simulink model "Ser_RLC_Sys"  (R2015a)
settings: Solver=ode23  StartTime=0.0  StopTime=0.01  RelTol=1e-3
settings Model: Creator=Kunal  LastModifiedBy=Kunal
settings SolverCC: AutoInsertRateTranBlk=on

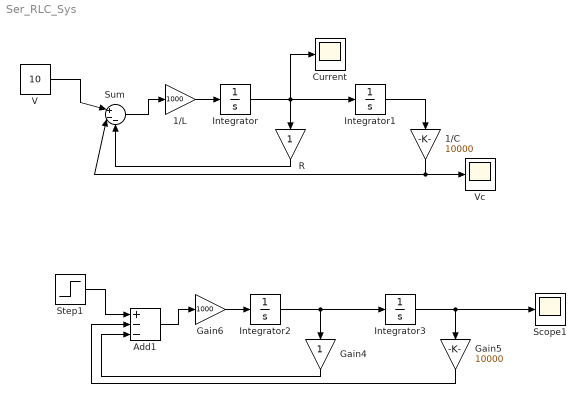
== system Ser_RLC_Sys ==
  1/C : Gain  Gain=10000
  1/L : Gain  Gain=1000
  Add1 : Sum  Inputs=+--
  Current : Scope
      settings: SaveName=ScopeData2  MaxDataPoints=5000000
  Gain4 : Gain
  Gain5 : Gain  Gain=10000
  Gain6 : Gain  Gain=1000
  Integrator{,1..3} (4 alike) : Integrator
  R : Gain
  Scope1 : Scope
  Step1 : Step  Time=0  After=10  SampleTime=0
  Sum : Sum  Inputs=|+--
  V : Constant  Value=10
  Vc : Scope
      settings: MaxDataPoints=5000000
  wires:
  Integrator/1 -> Current/1, Integrator1/1, R/1
  Integrator1/1 -> 1/C/1
  R/1 -> Sum/3
  Sum/1 -> 1/L/1
  V/1 -> Sum/1
  1/L/1 -> Integrator/1
  1/C/1 -> Sum/2, Vc/1
  Integrator2/1 -> Integrator3/1, Gain4/1
  Integrator3/1 -> Scope1/1, Gain5/1
  Gain4/1 -> Add1/3
  Add1/1 -> Gain6/1
  Step1/1 -> Add1/1
  Gain6/1 -> Integrator2/1
  Gain5/1 -> Add1/2
